simulink model "z2"  (R2017b)
settings: Solver=FixedStepDiscrete  StartTime=0.0  StopTime=0  RelTol=1e-3
undefined symbols (not defined in the file or in its folder): W
libraries: CPOiS_SourcesSinks x15, CPOiS_LinearTransforms x5
settings Model: Creator=alis  LastModifiedBy=alis

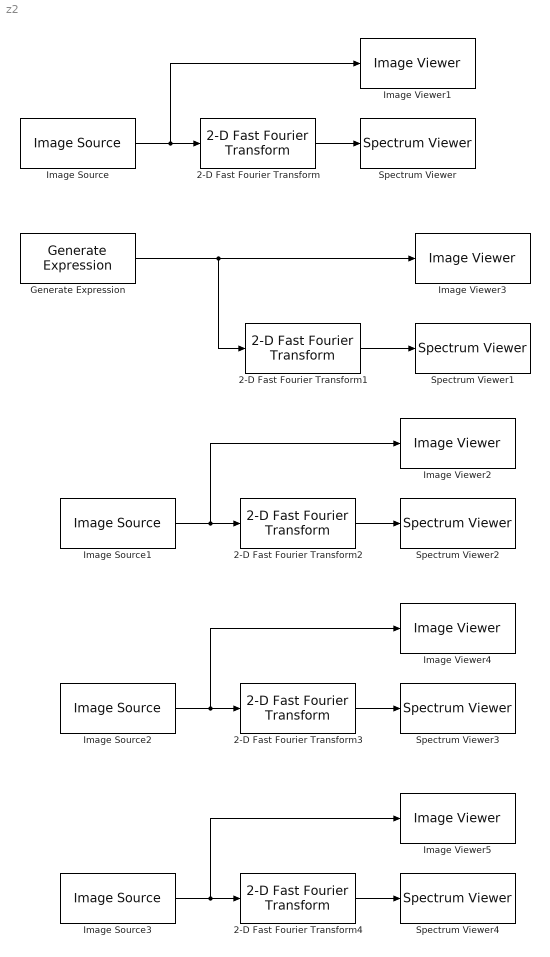
== system z2 ==
  2-D Fast Fourier Transform{,1..4} (5 alike) : CPOiS_LinearTransforms/2-D Fast Fourier Transform
      settings: SourceProductName=CPOiS - Digital image and signal processing
  Generate Expression : CPOiS_SourcesSinks/Generate Expression  Width=256  Height=256  Expression=128.*(sin(W)+1)
      settings: SourceProductName=CPOiS - Digital image and signal processing
  Image Source : CPOiS_SourcesSinks/Image Source  FileSelection=marine.png
      settings: SourceProductName=CPOiS - Digital image and signal processing
  Image Source1 : CPOiS_SourcesSinks/Image Source  FileSelection=rice.png
      settings: SourceProductName=CPOiS - Digital image and signal processing
  Image Source2 : CPOiS_SourcesSinks/Image Source  FileSelection=ball.png
      settings: SourceProductName=CPOiS - Digital image and signal processing
  Image Source3 : CPOiS_SourcesSinks/Image Source  FileSelection=cameraman.tif
      settings: SourceProductName=CPOiS - Digital image and signal processing
  Image Viewer{1..5} (5 alike) : CPOiS_SourcesSinks/Image Viewer
      settings: SourceProductName=CPOiS - Digital image and signal processing
  Spectrum Viewer{,1..4} (5 alike) : CPOiS_SourcesSinks/Spectrum Viewer
      settings: SourceProductName=CPOiS - Digital image and signal processing
  wires:
  Image Source/1 -> Image Viewer1/1, 2-D Fast Fourier Transform/1
  2-D Fast Fourier Transform/1 -> Spectrum Viewer/1
  2-D Fast Fourier Transform1/1 -> Spectrum Viewer1/1
  Generate Expression/1 -> Image Viewer3/1, 2-D Fast Fourier Transform1/1
  2-D Fast Fourier Transform2/1 -> Spectrum Viewer2/1
  Image Source1/1 -> Image Viewer2/1, 2-D Fast Fourier Transform2/1
  2-D Fast Fourier Transform3/1 -> Spectrum Viewer3/1
  Image Source2/1 -> Image Viewer4/1, 2-D Fast Fourier Transform3/1
  2-D Fast Fourier Transform4/1 -> Spectrum Viewer4/1
  Image Source3/1 -> Image Viewer5/1, 2-D Fast Fourier Transform4/1
